simulink model "A3_Publication"  (R2022a)
settings: Solver=FixedStepAuto  StartTime=0.0  StopTime=inf  FixedStep=0.1  RelTol=1e-3
model workspace (MAT data in the model file):
  SL_ROS_VariableLengthArrays_MaxSizes.CommonInfo.ArrayTruncateAction = 'EmitWarning'
  SL_ROS_VariableLengthArrays_MaxSizes.MsgTypeMap = containers.Map
  SL_ROS_VariableLengthArrays_MaxSizes.MsgTypeMap.serialization.keys = {'sensor_msgs/Image', 'sensor_msgs/LaserScan'}
  SL_ROS_VariableLengthArrays_MaxSizes.MsgTypeMap.serialization.values{1}(1).PropertyName = 'Data'
  SL_ROS_VariableLengthArrays_MaxSizes.MsgTypeMap.serialization.values{1}(1).DataType = 'uint8'
  SL_ROS_VariableLengthArrays_MaxSizes.MsgTypeMap.serialization.values{1}(1).MaxLength = 921600
  SL_ROS_VariableLengthArrays_MaxSizes.MsgTypeMap.serialization.values{1}(2).PropertyName = 'Encoding'
  SL_ROS_VariableLengthArrays_MaxSizes.MsgTypeMap.serialization.values{1}(2).DataType = 'uint8'
  SL_ROS_VariableLengthArrays_MaxSizes.MsgTypeMap.serialization.values{1}(2).MaxLength = 128
  SL_ROS_VariableLengthArrays_MaxSizes.MsgTypeMap.serialization.values{2}(1).PropertyName = 'Intensities'
  SL_ROS_VariableLengthArrays_MaxSizes.MsgTypeMap.serialization.values{2}(1).DataType = 'single'
  SL_ROS_VariableLengthArrays_MaxSizes.MsgTypeMap.serialization.values{2}(1).MaxLength = 128
  SL_ROS_VariableLengthArrays_MaxSizes.MsgTypeMap.serialization.values{2}(2).PropertyName = 'Ranges'
  SL_ROS_VariableLengthArrays_MaxSizes.MsgTypeMap.serialization.values{2}(2).DataType = 'single'
  SL_ROS_VariableLengthArrays_MaxSizes.MsgTypeMap.serialization.values{2}(2).MaxLength = 360
  SL_ROS_VariableLengthArrays_MaxSizes.MsgTypeMap.serialization.uniformity = 0
  SL_ROS_VariableLengthArrays_MaxSizes.MsgTypeMap.serialization.keyType = 'char'
  SL_ROS_VariableLengthArrays_MaxSizes.MsgTypeMap.serialization.valueType = 'any'
values from neighbouring files (symbols this model uses):
  WList = [0, 0, 0 ... (first row only)    [A1_WayAndObj.m]    (also in A1_WayDefAndObjSpawn.m; WList.mat = [0 6 3 9 12 15 18 0 0 6 9 0 ... (21 elements, 7x3)])
undefined symbols (not defined in the file or in its folder): Angular, gray, Linear, Rec, SDTV
libraries: robotlib x7, simulink x3, visiontextngfix x2, visionstatistics x2, visionconversions x1
settings Model: Creator=jacopo  LastModifiedBy=jacopo
settings OptimizationCC: EnhancedBackFolding=on  PassReuseOutputArgsAs=Individual arguments  ZeroExternalMemoryAtStartup=off  ZeroInternalMemoryAtStartup=off  MaxStackSize=64  OptimizeBlockOrder=speed  DifferentSizesBufferReuse=on  OptimizationCustomize=off  EfficientTunableParamExpr=on
settings DebuggingCC: ParameterTunabilityLossMsg=error
settings HardwareCC: ProdBitPerPointer=32  ProdBitPerSizeT=32  ProdBitPerPtrDiffT=32  ProdLargestAtomicFloat=None  ProdIntDivRoundTo=Undefined  ProdEndianess=Unspecified  ProdWordSize=32  ProdHWDeviceType=Generic->Unspecified (assume 32-bit Generic)
settings SFSimCC: MATLABDynamicMemAlloc=off
settings RTWCC: SystemTargetFile=ert.tlc  HardwareBoard=Robot Operating System (ROS)  TLCOptions="-aInlineSetEventsForThisBaseRateFcn=TLC_FALSE -aSuppressMultiTaskScheduler=TLC_FALSE  -aRateBasedStepFcn=0"  TemplateMakefile=ert_default_tmf  Toolchain=Catkin  TargetLang=C++
settings CodeAppCC: ForceParamTrailComments=on  IgnoreCustomStorageClasses=off  OperatorAnnotations=on  SimulinkDataObjDesc=on  SFDataObjDesc=on  InsertBlockDesc=on

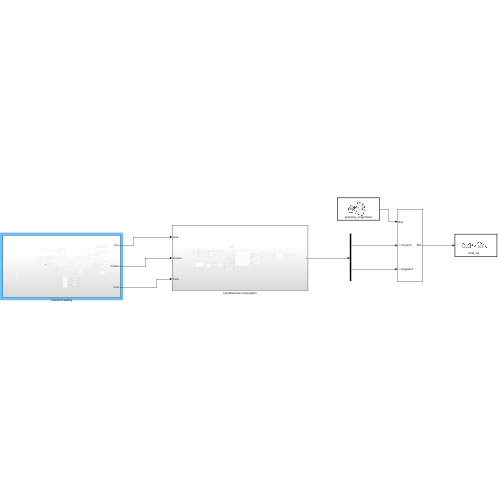
[thumbnail: Simulink's stored preview of the top-level diagram]
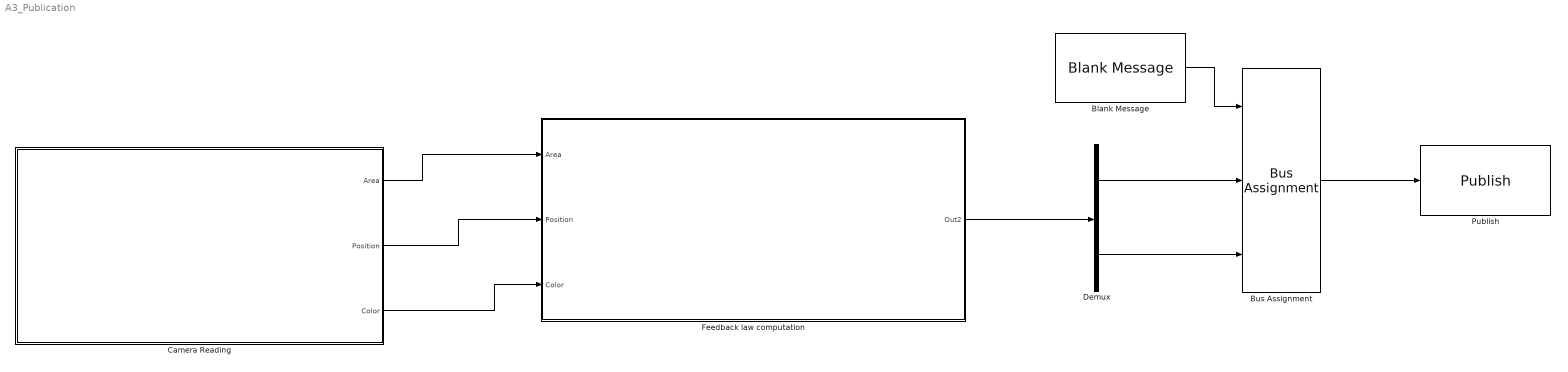
== system A3_Publication ==
  Blank Message : robotlib/Blank Message  messageClass=Message  entityType=geometry_msgs/Twist  messageType=geometry_msgs/Twist  SampleTime=inf  legacyBusStruct=off
  Bus Assignment : BusAssignment  AssignedSignals=Linear.X,Angular.Z
  Camera Reading : Subsystem
  Demux : Demux  Outputs=2
  Feedback law computation : Subsystem
  Publish : robotlib/Publish  topicSource=Select from ROS network  topic=/cmd_vel  messageType=geometry_msgs/Twist  legacyBusStruct=off  messageQueueLength=1
  wires:
  Demux/1 -> Bus Assignment/2
  Blank Message/1 -> Bus Assignment/1
  Demux/2 -> Bus Assignment/3
  Bus Assignment/1 -> Publish/1
  Feedback law computation/1(Out2) -> Demux/1
  Camera Reading/3(Color) -> Feedback law computation/3(Color)
  Camera Reading/2(Position) -> Feedback law computation/2(Position)
  Camera Reading/1(Area) -> Feedback law computation/1(Area)

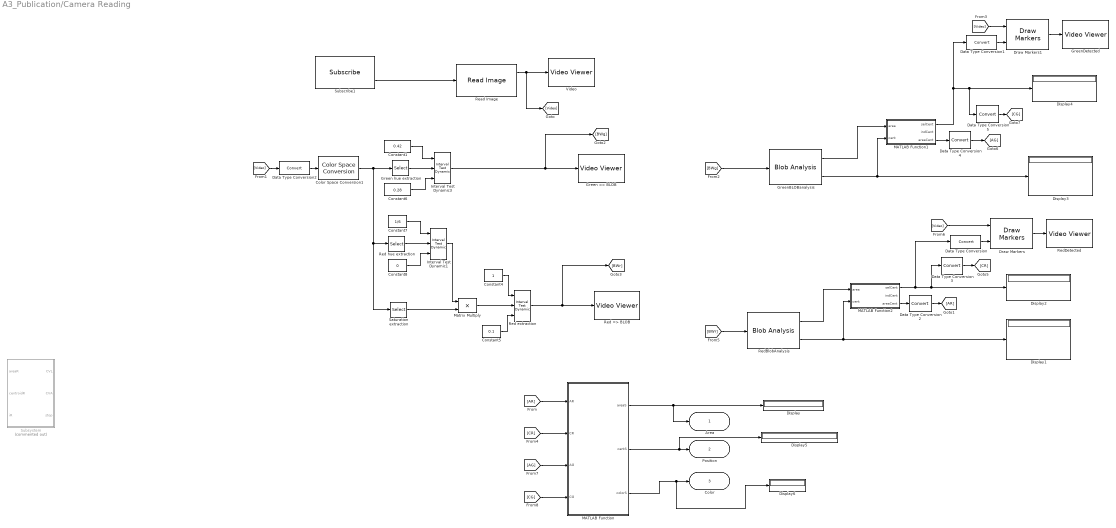
== system A3_Publication/Camera Reading ==
  Color Space Conversion1 : visionconversions/Color Space  Conversion  conversion=Obsolete  conversionActive=R'G'B' to HSV  wp_str=D65  rec=Rec. 601 (SDTV)  sys=1125/60/2:1  imagePorts=One multidimensional signal
  Constant1 : Constant  Value=0.42
  Constant4 : Constant
  Constant5 : Constant  Value=0.1
  Constant6 : Constant  Value=0.28
  Constant7 : Constant  Value=1/6
  Constant8 : Constant  Value=0
  Data Type Conversion{,1..2,2..5} (7 alike) : DataTypeConversion  SaturateOnIntegerOverflow=off  RndMeth=Floor
  Display{,1..6} (7 alike) : Display
  Draw Markers : visiontextngfix/Draw Markers  shape=Star  size=30  fill=off  fillClrSource=Specify via dialog  display=User-specified value  intensity=200  color=[255 0 0]  opacity=0.6  viewport=Entire image  antialiasing=off  inType=Obsolete  imagePorts=One multidimensional signal  roundingMode=Floor  overflowMode=off  memoryMode=Specify word length  memoryWordLength=16  memoryFracLength=15  prodOutputMode=Binary point scaling  prodOutputWordLength=32  prodOutputFracLength=14
      settings: SourceProductBaseCode=VP
  Draw Markers1 : visiontextngfix/Draw Markers  shape=Plus  size=30  fill=off  fillClrSource=Specify via dialog  display=User-specified value  intensity=200  color=[255 0 0]  opacity=0.6  viewport=Entire image  antialiasing=off  inType=Obsolete  imagePorts=One multidimensional signal  roundingMode=Floor  overflowMode=off  memoryMode=Specify word length  memoryWordLength=16  memoryFracLength=15  prodOutputMode=Binary point scaling  prodOutputWordLength=32  prodOutputFracLength=14
      settings: SourceProductBaseCode=VP
  Green => BLOB : VideoViewer  colormapValue=gray(256)  FigPos=[940 1078 591 337]
  Green hue extraction : Selector  NumberOfDimensions=3  InputPortWidth=3  IndexOptions=Index vector (dialog),Index vector (dialog),Index vector (dialog)  Indices=[1:480],[1:640],1  OutputSizes=1,1,1
  GreenBLOBanalysis : visionstatistics/Blob Analysis  Tag=vipblks_row_conv  area=on  centroid=on  bBox=off  majorAxis=off  minorAxis=off  angle=off  eccentricity=off  equivDiameterSq=off  extent=off  perimeter=off  outDT=double  conn=8  isLabel=off  maxBlobs=3  warnIfNumBlobsExceeded=on  isCount=off  useMinArea=off  minArea=0  useMaxArea=off  maxArea=intmax('uint32')  excludeBorderBlob=off  isOutVarDim=off  isFill=on  fillValues=-1  roundingMode=Floor  overflowMode=off  prodOutputMode=Binary point scaling  prodOutputWordLength=32  prodOutputFracLength=16  accumMode=Binary point scaling  accumWordLength=32  accumFracLength=0  outputMode=Binary point scaling  outputWordLength=32  outputFracLength=16  firstCoeffMode=Binary point scaling  firstCoeffWordLength=16  firstCoeffFracLength=14  secondCoeffMode=Binary point scaling  secondCoeffWordLength=32  secondCoeffFracLength=16
  GreenDetected : VideoViewer  colormapValue=gray(256)  FigPos=[854 1078 613 342]
  Interval Test Dynamic1 : simulink/Logic and Bit Operations/Interval Test Dynamic  IntervalClosedRight=on  IntervalClosedLeft=on  OutDataTypeStr=boolean
      settings: SourceProductBaseCode=SL
  Interval Test Dynamic3 : simulink/Logic and Bit Operations/Interval Test Dynamic  IntervalClosedRight=on  IntervalClosedLeft=on  OutDataTypeStr=boolean
      settings: SourceProductBaseCode=SL
  MATLAB Function : MATLAB Function  TreatAsAtomicUnit=on
  MATLAB Function1 : MATLAB Function  TreatAsAtomicUnit=on
  MATLAB Function2 : MATLAB Function  TreatAsAtomicUnit=on
  Matrix Multiply : Product
  Read Image : robotlib/Read Image  MaximumImageSize=[480, 640]  ImageEncoding=rgb8  ShowAlphaOutput=off  ShowErrorCodeOutput=on  VariableSizeOutputs=off
      settings: SourceProductBaseCode=RR
  Red => BLOB : VideoViewer  colormapValue=gray(256)  FigPos=[714 828 561 358]
  Red extraction : simulink/Logic and Bit Operations/Interval Test Dynamic  IntervalClosedRight=on  IntervalClosedLeft=on  OutDataTypeStr=boolean
      settings: SourceProductBaseCode=SL
  Red hue extraction : Selector  NumberOfDimensions=3  InputPortWidth=3  IndexOptions=Index vector (dialog),Index vector (dialog),Index vector (dialog)  Indices=[1:480],[1:640],1  OutputSizes=1,1,1
  RedBlobAnalysis : visionstatistics/Blob Analysis  Tag=vipblks_row_conv  area=on  centroid=on  bBox=off  majorAxis=off  minorAxis=off  angle=off  eccentricity=off  equivDiameterSq=off  extent=off  perimeter=off  outDT=double  conn=8  isLabel=off  maxBlobs=3  warnIfNumBlobsExceeded=on  isCount=off  useMinArea=off  minArea=0  useMaxArea=off  maxArea=intmax('uint32')  excludeBorderBlob=off  isOutVarDim=off  isFill=on  fillValues=-1  roundingMode=Floor  overflowMode=off  prodOutputMode=Binary point scaling  prodOutputWordLength=32  prodOutputFracLength=16  accumMode=Binary point scaling  accumWordLength=32  accumFracLength=0  outputMode=Binary point scaling  outputWordLength=32  outputFracLength=16  firstCoeffMode=Binary point scaling  firstCoeffWordLength=16  firstCoeffFracLength=14  secondCoeffMode=Binary point scaling  secondCoeffWordLength=32  secondCoeffFracLength=16
  RedDetected : VideoViewer  colormapValue=gray(256)  FigPos=[1085 1035 593 356]
  Saturation extraction : Selector  NumberOfDimensions=3  InputPortWidth=3  IndexOptions=Index vector (dialog),Index vector (dialog),Index vector (dialog)  Indices=[1:480],[1:640],2  OutputSizes=1,1,1
  Subscribe1 : robotlib/Subscribe  topicSource=Select from ROS network  topic=/camera/rgb/image_raw  messageType=sensor_msgs/Image  SampleTime=-1  legacyBusStruct=off  messageQueueLength=1
  Subsystem : Subsystem  Commented=on
  Video : VideoViewer  colormapValue=gray(256)  FigPos=[689 794 566 352]
  Area : Outport
  Position : Outport  Port=2
  Color : Outport  Port=3
  wires:
  Subscribe1/2 -> Read Image/1
  Constant7/1 -> Interval Test Dynamic1/1
  Read Image/1 -> [Video], Video/1
  Saturation extraction/1 -> Matrix Multiply/2
  Color Space Conversion1/1 -> Green hue extraction/1, Saturation extraction/1, Red hue extraction/1
  [Video] -> Data Type Conversion2/1
  Constant4/1 -> Red extraction/1
  Constant5/1 -> Red extraction/3
  Red hue extraction/1 -> Interval Test Dynamic1/2
  Red extraction/1 -> [BWr], Red => BLOB/1
  Matrix Multiply/1 -> Red extraction/2
  Interval Test Dynamic1/1 -> Matrix Multiply/1
  Constant8/1 -> Interval Test Dynamic1/3
  Data Type Conversion2/1 -> Color Space Conversion1/1
  Green hue extraction/1 -> Interval Test Dynamic3/2
  Constant6/1 -> Interval Test Dynamic3/3
  Constant1/1 -> Interval Test Dynamic3/1
  Interval Test Dynamic3/1 -> [BWg], Green => BLOB/1
  [BWr] -> RedBlobAnalysis/1
  RedBlobAnalysis/2 -> Display1/1, MATLAB Function2/2(cent)
  Draw Markers/1 -> RedDetected/1
  Data Type Conversion/1 -> Draw Markers/2
  [Video] -> Draw Markers/1
  RedBlobAnalysis/1 -> MATLAB Function2/1(area)
  MATLAB Function2/1(selCent) -> Data Type Conversion3/1, Display2/1, Data Type Conversion/1
  GreenBLOBanalysis/1 -> MATLAB Function1/1(area)
  MATLAB Function1/1(selCent) -> Data Type Conversion1/1, Data Type Conversion5/1, Display4/1
  [Video] -> Draw Markers1/1
  Data Type Conversion1/1 -> Draw Markers1/2
  Draw Markers1/1 -> GreenDetected/1
  GreenBLOBanalysis/2 -> Display3/1, MATLAB Function1/2(cent)
  [BWg] -> GreenBLOBanalysis/1
  MATLAB Function/2(centS) -> Display5/1, Position/1
  MATLAB Function/3(colorS) -> Display6/1, Color/1
  [AR] -> MATLAB Function/1(AR)
  [CR] -> MATLAB Function/2(CR)
  [AG] -> MATLAB Function/3(AG)
  [CG] -> MATLAB Function/4(CG)
  MATLAB Function2/3(areaCent) -> Data Type Conversion2/1
  Data Type Conversion2/1 -> [AR]
  Data Type Conversion3/1 -> [CR]
  MATLAB Function1/3(areaCent) -> Data Type Conversion4/1
  Data Type Conversion4/1 -> [AG]
  Data Type Conversion5/1 -> [CG]
  MATLAB Function/1(areaS) -> Display/1, Area/1

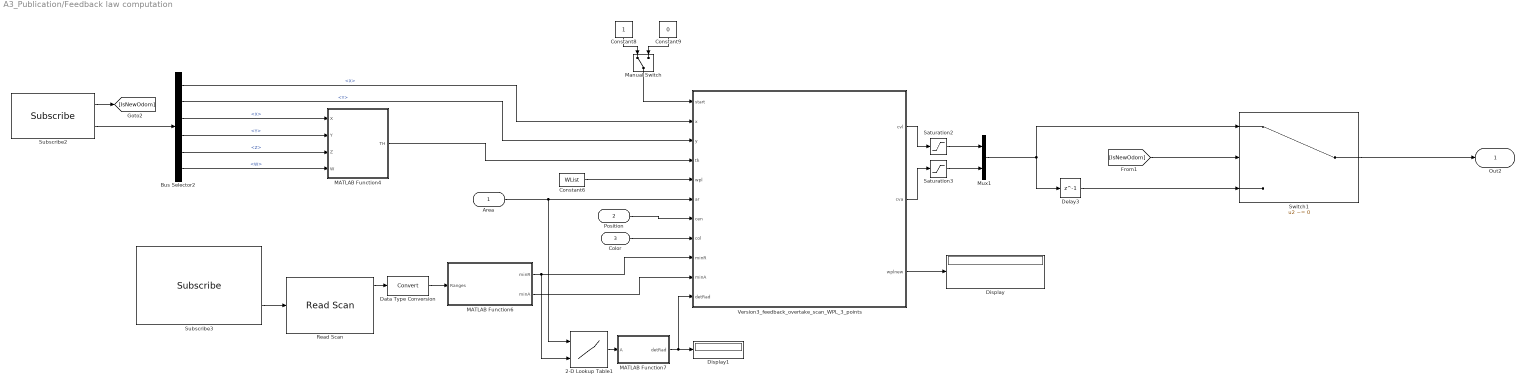
== system A3_Publication/Feedback law computation ==
  Area : Inport
  Position : Inport  Port=2
  Color : Inport  Port=3
  2-D Lookup Table1 : Lookup_n-D  BreakpointsForDimension1=[4220 10400 45519 96000]  BreakpointsForDimension2=[0.5 0.8 1.8 2.8]  Table=[0.00400713348672168 0.0102582617260075 0.0519324499879129 0.125663706143592;0.00969627362219072 0.0248224604728083 0.125663706143592 0.304075140791901;0.0490873852123405 0.125663706143592 0.636172512351933 1.539380400259;0.125663706143592 0.321699087727595 1.62860163162095 3.94081382466304]  InternalRulePriority=Speed  RndMeth=Simplest
      settings: InputPortMap=u0,u1
  Bus Selector2 : BusSelector  OutputSignals=Pose.Pose.Position.X,Pose.Pose.Position.Y,Pose.Pose.Orientation.X,Pose.Pose.Orientation.Y,Pose.Pose.Orientation.Z,Pose.Pose.Orientation.W
  Constant6 : Constant  Value=WList
  Constant8 : Constant
  Constant9 : Constant  Value=0
  Data Type Conversion : DataTypeConversion  SaturateOnIntegerOverflow=off  RndMeth=Floor
  Delay3 : Delay  DelayLength=1
  Display : Display
  Display1 : Display
  MATLAB Function4 : MATLAB Function  TreatAsAtomicUnit=on
  MATLAB Function6 : MATLAB Function  TreatAsAtomicUnit=on
  MATLAB Function7 : MATLAB Function  TreatAsAtomicUnit=on
  Manual Switch : ManualSwitch
  Mux1 : Mux  Inputs=2
  Read Scan : robotlib/Read Scan  MaximumArrayLength=360  ShowAnglesOutput=on  ShowIntensityOutput=off  ShowErrorCodeOutput=on  VariableSizeOutputs=off
      settings: SourceProductBaseCode=RR
  Saturation2 : Saturate  UpperLimit=0.2  LowerLimit=-0.2
  Saturation3 : Saturate  UpperLimit=0.4  LowerLimit=-0.4
  Subscribe2 : robotlib/Subscribe  topicSource=Select from ROS network  topic=/odom  messageType=nav_msgs/Odometry  SampleTime=-1  legacyBusStruct=off  messageQueueLength=1
  Subscribe3 : robotlib/Subscribe  topicSource=Select from ROS network  topic=/scan  messageType=sensor_msgs/LaserScan  SampleTime=-1  legacyBusStruct=off  messageQueueLength=1
  Switch1 : Switch  Criteria=u2 ~= 0  SaturateOnIntegerOverflow=off  InputSameDT=off
  Version3_feedback_overtake_scan_WPL_3_points : Stateflow chart  TreatAsAtomicUnit=on
  Out2 : Outport
  wires:
  Color/1 -> Version3_feedback_overtake_scan_WPL_3_points/8(col)
  Position/1 -> Version3_feedback_overtake_scan_WPL_3_points/7(cen)
  Area/1 -> 2-D Lookup Table1/1, Version3_feedback_overtake_scan_WPL_3_points/6(ar)
  Constant6/1 -> Version3_feedback_overtake_scan_WPL_3_points/5(wpl)
  Bus Selector2/1 -> Version3_feedback_overtake_scan_WPL_3_points/2(x)  "<X>"
  Bus Selector2/6 -> MATLAB Function4/4(W)  "<W>"
  MATLAB Function4/1(TH) -> Version3_feedback_overtake_scan_WPL_3_points/4(th)
  Bus Selector2/5 -> MATLAB Function4/3(Z)  "<Z>"
  Subscribe2/1 -> [IsNewOdom]
  Bus Selector2/3 -> MATLAB Function4/1(X)  "<X>"
  Subscribe2/2 -> Bus Selector2/1
  Bus Selector2/2 -> Version3_feedback_overtake_scan_WPL_3_points/3(y)  "<Y>"
  Bus Selector2/4 -> MATLAB Function4/2(Y)  "<Y>"
  Manual Switch/1 -> Version3_feedback_overtake_scan_WPL_3_points/1(start)
  Constant8/1 -> Manual Switch/1
  Constant9/1 -> Manual Switch/2
  Saturation2/1 -> Mux1/1
  Switch1/1 -> Out2/1
  Version3_feedback_overtake_scan_WPL_3_points/2(cva) -> Saturation3/1
  Version3_feedback_overtake_scan_WPL_3_points/1(cvl) -> Saturation2/1
  [IsNewOdom] -> Switch1/2
  Saturation3/1 -> Mux1/2
  Mux1/1 -> Switch1/1, Delay3/1
  Delay3/1 -> Switch1/3
  Subscribe3/2 -> Read Scan/1
  Read Scan/1 -> Data Type Conversion/1
  Data Type Conversion/1 -> MATLAB Function6/1(Ranges)
  MATLAB Function6/1(minR) -> 2-D Lookup Table1/2, Version3_feedback_overtake_scan_WPL_3_points/9(minR)
  MATLAB Function6/2(minA) -> Version3_feedback_overtake_scan_WPL_3_points/10(minA)
  MATLAB Function7/1(detRad) -> Display1/1, Version3_feedback_overtake_scan_WPL_3_points/11(detRad)
  Version3_feedback_overtake_scan_WPL_3_points/3(wplnew) -> Display/1
  2-D Lookup Table1/1 -> MATLAB Function7/1(A)

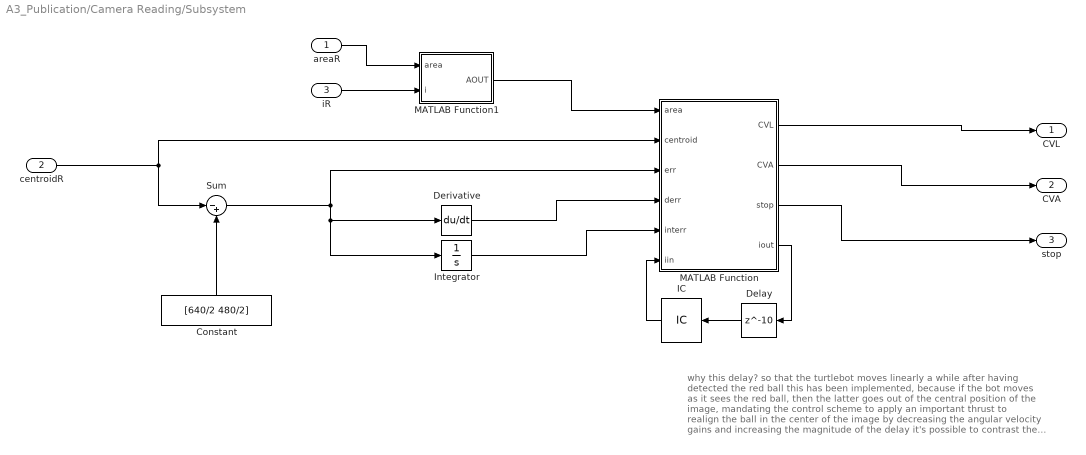
== system A3_Publication/Camera Reading/Subsystem ==
  note: why this delay? so that the turtlebot moves linearly a while after
      | having detected the red ball
      | this has been implemented, because if the bot moves as it sees
      | the red ball, then the latter goes out of the central position of the image,
      | mandating the control scheme to apply an important thrust to realign
      | the ball in the center of the image
      | by decreasing the angular velocity gains and increasing the magnitude
      | of the delay it's possible to contrast the wobbly motion, caused by
      | a synergic cooperation of high gains and moving linearly too early
  areaR : Inport
  centroidR : Inport  Port=2
  iR : Inport  Port=3
  Constant : Constant  Value=[640/2 480/2]  VectorParams1D=off
  Delay : Delay  DelayLength=10
  Derivative : Derivative
  IC : InitialCondition  Value=0
  Integrator : Integrator
  MATLAB Function : MATLAB Function  TreatAsAtomicUnit=on
  MATLAB Function1 : MATLAB Function  TreatAsAtomicUnit=on
  Sum : Sum  Inputs=|-+
  CVL : Outport
  CVA : Outport  Port=2
  stop : Outport  Port=3
  wires:
  MATLAB Function/3(stop) -> stop/1
  areaR/1 -> MATLAB Function1/1(area)
  MATLAB Function/2(CVA) -> CVA/1
  MATLAB Function/1(CVL) -> CVL/1
  MATLAB Function1/1(AOUT) -> MATLAB Function/1(area)
  iR/1 -> MATLAB Function1/2(i)
  centroidR/1 -> Sum/1, MATLAB Function/2(centroid)
  Constant/1 -> Sum/2
  Sum/1 -> Integrator/1, Derivative/1, MATLAB Function/3(err)
  Derivative/1 -> MATLAB Function/4(derr)
  Integrator/1 -> MATLAB Function/5(interr)
  Delay/1 -> IC/1
  MATLAB Function/4(iout) -> Delay/1
  IC/1 -> MATLAB Function/6(iin)

== matlab function A3_Publication/Camera Reading/MATLAB Function1 ==
  data: area input; cent input; selCent output; indCent output; areaCent output
function [selCent, indCent, areaCent]  = fcn(area,cent)

[areaCent, indCent] = max(area);

if ~isempty(indCent)
    selCent = cent(indCent,:);
else 
    selCent = [0,0];
end

== matlab function A3_Publication/Camera Reading/Subsystem/MATLAB Function ==
  data: area input; CVL output; centroid input; CVA output; err input; stop output; derr input; interr input; iin input; iout output
function [CVL, CVA, stop, iout] = fcn(area, centroid, err, derr, interr, iin)

NC = 2; % max number of centroids
NoCV = - ones(NC, 2);

if centroid == NoCV
    CVL = 0;
    CVA = 0.2;
    iout = 0; %add
else
    iout = 1; %add
    kPL = 0.05;
%     kPA = 0.1;
%     kPA = 0.01;
    kPA = 0.003; % 0.01 is too high % 0.005 mmmh almost
    kDA = 0.01*0;
    kIA = 0;
    
    ERR = err(1);
    dERR = derr(1);
    intERR = interr(1);

    if iin == 1  %add
        CVL = kPL*area;
    else
        CVL = 0;
    end

    CVA = kPA*ERR + kDA*dERR + kIA*intERR;
end

maxA = 0.9*(640*480);

if area < maxA
    stop = 0;
else
    CVL = 0;
    CVA = 0;
    stop = 1;
end


% % centroidsel = centroid( centroid ~= [-1 -1])'; % not that robust

== matlab function A3_Publication/Camera Reading/MATLAB Function2 ==
  data: area input; cent input; selCent output; indCent output; areaCent output
function [selCent, indCent, areaCent]  = fcn(area,cent)

[areaCent, indCent] = max(area);

if ~isempty(indCent)
    selCent = cent(indCent,:);
else 
    selCent = [0,0];
end

== matlab function A3_Publication/Camera Reading/Subsystem/MATLAB Function1 ==
  data: area input; AOUT output; i input
function AOUT = fcn(area, i)

AOUT = area(i, 1);

== matlab function A3_Publication/Camera Reading/MATLAB Function ==
  data: AR input; CR input; areaS output; centS output; colorS output; AG input; CG input
function [areaS, centS, colorS] = fcn(AR, CR, AG, CG)

% 1 is red, 2 is green, 0 is none

if AR > AG
    areaS = AR;
    centS = CR;
    colorS = 1;
elseif AR < AG
    areaS = AG;
    centS = CG;
    colorS = 2;
else
    areaS = 0;
    centS = [0 0];
    colorS = 0;
end

== stateflow chart A3_Publication/Feedback law computation/Version3_feedback_overtake_scan_WPL_3_points ==
  note: alternative to Final Project 2: the cvlFixed can be avoided
  state Still
    cvl = 0;
    cva = 0;
    index = 1;
    kPL = 0.48;
    kPA = 2.2;
    overT = 1;
  state Overtaking
    [Dist, ErrTh, overT] = OTdisterrfun(x, y, th, wplnew, overT);
    cva = kPA*ErrTh;
  state FBMotion
    [Dist, ErrTh] = disterrfun(x, y, th, wpl, index);
    cvl = kPL*Dist;
    cva = kPA*ErrTh;
  state Stop
    cvl = 0;
    cva = 0;
  state Turning
    [Dist, ErrTh] = disterrfun(x, y, th, wpl, index);
    cvl = 0;
    cva = (0.9*kPA)*ErrTh;
  Still -> FBMotion [order 2] : [start == 1]
  FBMotion -> Overtaking [order 2] : [minR <= 0.8 && (350 < minA || minA < 10)] {wplnew = OTlist(detRad, minR, x, y, th, col)}
  (default) -> Still
  FBMotion -> FBMotion [order 4] : [Dist > 0.05]
  Still -> Still [order 1] : [start == 0]
  Overtaking -> Overtaking [order 1] : [Dist <= 0.2 && overT < 3]{overT = overT + 1}
  Overtaking -> FBMotion [order 2] : [Dist <= 0.2 && overT == 3]{overT = 1}
  FBMotion -> Stop [order 1] : [index == length(wpl) + 1]
  Turning -> FBMotion [order 3] : [abs(ErrTh) <= 0.05] {index = index + 1}
  FBMotion -> Turning [order 3] : [Dist <= 0.05 ]
  Turning -> Stop [order 1] : [abs(ErrTh) <= 0.05 && index == length(wpl) ]
  Turning -> Turning [order 2] : [abs(ErrTh) > 0.05]
  data: X function_input; Y function_input; Th function_input; WPL function_input; dist function_output; errTh function_output; IND function_input; detrad function_input; MINR function_input; WPLN function_output; X function_input; Y function_input; Th function_input; COL function_input; dist function_output; errTh function_output; X function_input; Y function_input; Th function_input; WPLN function_input; OT function_input; OT function_output; start input; x input; y input; th input; wpl input; ar input; cen input; col input; Dist local; ErrTh local; cvl output; cva output; index local; kPA local; kPL local; overT local; minR input; minA input; detRad input; wplnew output; cvlFixed local
  function [dist, errTh] = disterrfun(X, Y, Th, WPL, IND):
    | function [dist, errTh] = disterrfun(X, Y, Th, WPL, IND)
    |  
    | tol = 1e-2;
    | 
    | POSr = WPL(IND, :);
    | 
    | Xr = POSr(1); Yr = POSr(2); Thr = POSr(3);
    | 
    | if pi < Thr && Thr < 2*pi
    |     Thr = Thr - 2*pi;
    | end
    | 
    | Gr = Thr;
    | Z = (Xr - X) + 1i*(Yr - Y);
    | dist = abs(Z);
    | 
    | 
    | if dist <= 0.1
    |     if (Th > tol) && (- pi + tol < Gr && Gr < - pi/2 - tol)
    |         Gr = Gr + 2*pi;
    |     elseif (- pi + tol < Th && Th < - pi/2 - tol) && (Gr > tol)
    |         Th = Th + 2*pi;
    |     end
    | else
    |     Gr = angle(Z);
    |     if (Th > tol) && (- pi + tol < Gr && Gr < - pi/2 - tol)
    |         Gr = Gr + 2*pi;
    |     elseif (- pi + tol < Th && Th < - pi/2 - tol) && (Gr > tol)
    |         Th = Th + 2*pi;
    |     end
    | end
    | 
    | errTh = Gr - Th;
  function WPLN = OTlist(detrad, MINR, X, Y, Th, COL):
    | function WPLN = OTlist(detrad, MINR, X, Y, Th, COL)
    | Xa = 0.75*MINR;
    | Xb = Xa + 1.1*detrad;
    | 
    | if COL == 1
    |     Ya = 2*detrad/2;
    | else
    |     Ya = -2*detrad/2;
    | end
    | 
    | Yb = Ya;
    | 
    | xa = X + Xa*cos(Th) - Ya*sin(Th);
    | ya = Y + Xa*sin(Th) + Ya*cos(Th);
    | 
    | xb = X + Xb*cos(Th) - Yb*sin(Th);
    | yb = Y + Xb*sin(Th) + Yb*cos(Th);
    | 
    | L = 2*minR + 0.4*detrad;
    | 
    | xc = X + L*cos(Th);
    | yc = Y + L*sin(Th);
    | 
    | WPLN = [xa, ya; xb, yb; xc, yc];
    | 
    | end
  function [dist, errTh, OT] = OTdisterrfun(X, Y, Th, WPLN, OT):
    | function [dist, errTh, OT] = OTdisterrfun(X, Y, Th, WPLN, OT)
    | 
    | tol = 1e-2;
    | 
    | POSr = WPLN(OT, :);
    | 
    | Xr = POSr(1); Yr = POSr(2);
    | Z = (Xr - X) + 1i*(Yr - Y);
    | dist = abs(Z);
    | Gr = angle(Z);
    | 
    | if (Th > tol) && (- pi + tol < Gr && Gr < - pi/2 - tol)
    |     Gr = Gr + 2*pi;
    | elseif (- pi + tol < Th && Th < - pi/2 - tol) && (Gr > tol)
    |     Th = Th + 2*pi;
    | end
    | 
    | errTh = Gr - Th;
    | 
    | 
    | end

== matlab function A3_Publication/Feedback law computation/MATLAB Function4 ==
  data: X input; TH output; Y input; Z input; W input
function TH = fromQuat2Eu(X, Y, Z, W)



ANGLE = quat2eul([W, X, Y, Z]);

TH = ANGLE(1);

== matlab function A3_Publication/Feedback law computation/MATLAB Function6 ==
  data: minR output; Ranges input; minA output
function [minR, minA] = PlotAndMin(Ranges)

double minR
double minA

if any(Ranges > 0)
    [minR, minA] = min(Ranges);
else
    minR = -1;
    minA = -1;
end

end

== matlab function A3_Publication/Feedback law computation/MATLAB Function7 ==
  data: A input; detRad output
function detRad = fcn(A)
% despite the name, this outputs the detected diameter

detRad = 2*sqrt(abs(A)/pi);

end
